simulink model "modelForTest"  (R2021b)
settings: Solver=VariableStepAuto  StartTime=0.0  StopTime=1.0  RelTol=1e-3
model workspace (MATLAB code in the model file):
  | utils = StateMachineUtils;
  | 
  | utils = utils.loadEventsInAds('resources/tct/ALLEVENT.ADS');
  | utils = utils.createEventsTable();
  | 
  | utils = utils.loadDisabledEventsInPdt('resources/tct/DATA_SIMSUP1_MG1.PDT');
  | 
  | utils = utils.loadTransitionsInAds('resources/tct/SIMSUP1_MG1.ADS');
  | 
  | eventsTable = utils.getEventsTable();
  | eventsArray = eventsTable.event;
  | activeEvents = eventsTable.isActive;
  | 
  | switchedOffEvents = utils.getSwitchedOffEvents();
  | transitions = utils.getTransitions();
  | 
  | 
  | example.ex1 = [1 2 3 4];
  | example.ex2 = [1 2];
settings Model: Creator=raquelgrillo  LastModifiedBy=raquelgrillo

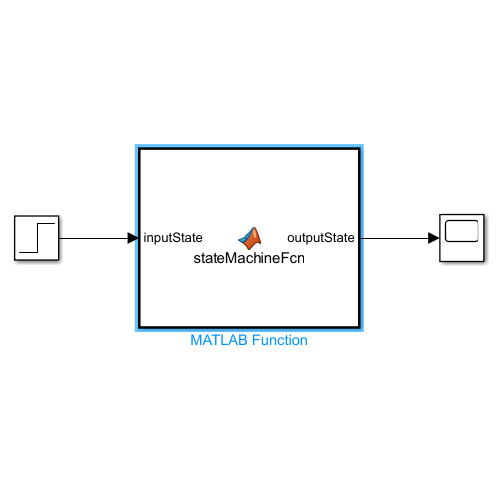
[thumbnail: Simulink's stored preview of the top-level diagram]
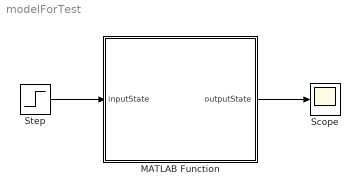
== system modelForTest ==
  MATLAB Function : MATLAB Function  TreatAsAtomicUnit=on
  Scope : Scope
  Step : Step  Time=0.5  SampleTime=0
  wires:
  Step/1 -> MATLAB Function/1(inputState)
  MATLAB Function/1(outputState) -> Scope/1

== matlab function modelForTest/MATLAB Function ==
  data: inputState input; outputState output; eventsArray parameter; example parameter; transitions parameter; activeEvents parameter
function outputState  = stateMachineFcn( ...
    inputState, ...
    eventsArray, ...
    example, ...
    transitions, ...
    activeEvents)
persistent stateMachine

if (isempty(stateMachine))
    
    stateMachine = StateMachine(eventsArray, activeEvents, example, transitions);
end

stateMachine = stateMachine.setState(inputState);
outputState = stateMachine.getCurrentState();
